simulink model "FxLMS_Sys"  (R2024b)
settings: Solver=FixedStepDiscrete  StartTime=0.0  StopTime=10  FixedStep=1/48000  RelTol=1e-3
values from neighbouring files (symbols this model uses):
  sim_p = conv(sim_s,sim_f)    [FxLMS_algo_sim.m]
  sim_s = [0.5 0.5 -0.3 -0.3 -0.2 -0.2]    [FxLMS_algo_sim.m]
undefined symbols (not defined in the file or in its folder): dspblkCoreblockFVToolHelper, gcbh
libraries: dspsrcs4 x2, dspadpt3 x1, dspfdesign x1
settings Model: PacingRate=10  Creator=shaar  LastModifiedBy=shaar

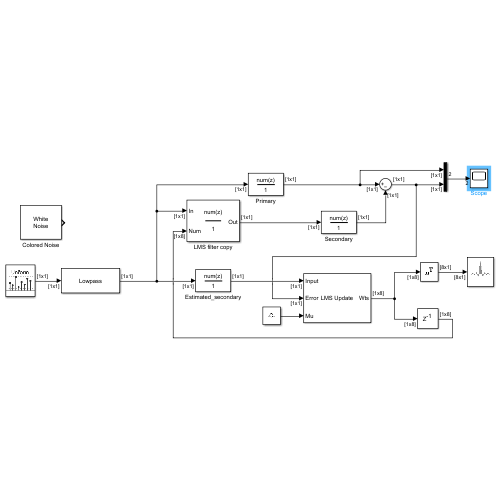
[thumbnail: Simulink's stored preview of the top-level diagram]
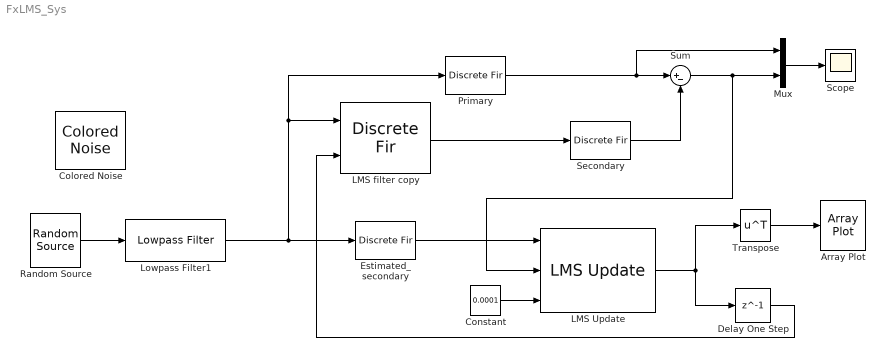
== system FxLMS_Sys ==
  Array Plot : ArrayPlot  WindowPosition=[49.000000,142.000000,800.000000,500.000000,]  ScopeFrameLocation=window  YLimits=[-0.0675 0.067]
  Colored Noise : dspsrcs4/Colored Noise  Color=white  InverseFrequencyPower=1  BoundedOutput=on  NumChannels=1  OutputDataType=double  SamplesPerFrame=1  SampleTime=1/48000  RandomStream=mt19937ar with seed  Seed=67  SimulateUsing=Interpreted execution
      settings: LibrarySourceBlock=audiosources/Colored Noise
  Constant : Constant  Value=0.0001
  Delay One Step : Delay  DelayLength=1
  Estimated_secondary : DiscreteFir  LoadFcn=dspblkCoreblockFVToolHelper(gcbh,'load');  Coefficients=sim_s
      settings: CopyFcn=dspblkCoreblockFVToolHelper(gcbh,'copy');  DeleteFcn=dspblkCoreblockFVToolHelper(gcbh,'close');  ModelCloseFcn=dspblkCoreblockFVToolHelper(gcbh,'close');  PreSaveFcn=dspblkCoreblockFVToolHelper(gcbh,'presave');  PostSaveFcn=dspblkCoreblockFVToolHelper(gcbh,'postsave');  CloseFcn=dspblkCoreblockFVToolHelper(gcbh,'close');
  LMS Update : dspadpt3/LMS Update  Method=Normalized LMS  Length=8  NumFilters=1  StepSizeSource=Input port  StepSize=0.1  LeakageFactor=1.0  InitialConditions=0  AdaptiveFilterMode=Tapped delay-line FIR filter  EnableAdaptInput=off  EnableResetInput=off  SimulateUsing=Interpreted execution
  LMS filter copy : DiscreteFir  LoadFcn=dspblkCoreblockFVToolHelper(gcbh,'load');  CoefSource=Input port
      settings: CopyFcn=dspblkCoreblockFVToolHelper(gcbh,'copy');  DeleteFcn=dspblkCoreblockFVToolHelper(gcbh,'close');  ModelCloseFcn=dspblkCoreblockFVToolHelper(gcbh,'close');  PreSaveFcn=dspblkCoreblockFVToolHelper(gcbh,'presave');  PostSaveFcn=dspblkCoreblockFVToolHelper(gcbh,'postsave');  CloseFcn=dspblkCoreblockFVToolHelper(gcbh,'close');  InputPortMap=u0,u1
  Lowpass Filter1 : dspfdesign/Lowpass Filter  FilterType=FIR  DesignForMinimumOrder=on  FilterOrder=50  PassbandFrequency=0.0125  StopbandFrequency=0.0167  PassbandRipple=0.1  StopbandAttenuation=80  SampleRateMode=Use normalized frequency (0 to 1)  SampleRate=44100  SimulateUsing=Interpreted execution  roundingMode=Floor  coeffsDataTypeStr=fixdt(1,16)
  Mux : Mux  Inputs=2
  Primary : DiscreteFir  LoadFcn=dspblkCoreblockFVToolHelper(gcbh,'load');  Coefficients=sim_p
      settings: CopyFcn=dspblkCoreblockFVToolHelper(gcbh,'copy');  DeleteFcn=dspblkCoreblockFVToolHelper(gcbh,'close');  ModelCloseFcn=dspblkCoreblockFVToolHelper(gcbh,'close');  PreSaveFcn=dspblkCoreblockFVToolHelper(gcbh,'presave');  PostSaveFcn=dspblkCoreblockFVToolHelper(gcbh,'postsave');  CloseFcn=dspblkCoreblockFVToolHelper(gcbh,'close');
  Random Source : dspsrcs4/Random Source  SrcType=Uniform  MinVal=-0.05  MaxVal=0.05  MeanVal=0  VarVal=1  RepMode=Specify seed  rawSeed=1  IsInherit=off  SampTime=1/48000  SampFrame=1  OutComplex=Real  DataType=double  SimulateUsing=Interpreted execution
  Scope : Scope
  Secondary : DiscreteFir  LoadFcn=dspblkCoreblockFVToolHelper(gcbh,'load');  Coefficients=sim_s
      settings: CopyFcn=dspblkCoreblockFVToolHelper(gcbh,'copy');  DeleteFcn=dspblkCoreblockFVToolHelper(gcbh,'close');  ModelCloseFcn=dspblkCoreblockFVToolHelper(gcbh,'close');  PreSaveFcn=dspblkCoreblockFVToolHelper(gcbh,'presave');  PostSaveFcn=dspblkCoreblockFVToolHelper(gcbh,'postsave');  CloseFcn=dspblkCoreblockFVToolHelper(gcbh,'close');
  Sum : Sum  Inputs=|+-
  Transpose : Math  Operator=transpose
  wires:
  Lowpass Filter1/1 -> Estimated_secondary/1, LMS filter copy/1, Primary/1
  Primary/1 -> Mux/1, Sum/1
  Secondary/1 -> Sum/2
  LMS filter copy/1 -> Secondary/1
  Sum/1 -> Mux/2, LMS Update/2
  LMS Update/1 -> Delay One Step/1, Transpose/1
  Delay One Step/1 -> LMS filter copy/2
  Transpose/1 -> Array Plot/1
  Constant/1 -> LMS Update/3
  Estimated_secondary/1 -> LMS Update/1
  Mux/1 -> Scope/1
  Random Source/1 -> Lowpass Filter1/1
